simulink model "Offline_DataImport_AND_ECGAnalysis_AND_SCGAnalysis"  (R2020b)
settings: Solver=FixedStepDiscrete  StartTime=0.0  StopTime=param_sim_time  FixedStep=1/fs  MaxStep=1/fs  RelTol=1e-3
undefined symbols (not defined in the file): analyses, fdesignblkfcn, fs, gcbh, param_tot_samples
libraries: dspstat3 x1
(part 5 of 5)

== matlab function Offline_DataImport_AND_ECGAnalysis_AND_SCGAnalysis/SCG Analysis/Enabled SCG Analysis Subsystem/Signal Generation/3D Projections/SCG xyz Average Cycle/Average SCGxyz Cycle Calculator ==
  data: r_pos input; scgxyz input; scgxyz_avgcycle output size=[3*fs 3]
function scgxyz_avgcycle  = slk_avg_scgxyz_cycle_calculator(r_pos,scgxyz)
% Simulink function to return the average x,y, and z cycles of the SCG.

% INPUTS:
% r_pos = index positions of the R peaks of the ecg.
% scgxyz = matrix of size [length_scg 3] with the (normally pre-processed) SCG
%          x,y, and z components. The first column corresponds to SCGx, the second
%          to SCGy and the third to SCGz.

% OUTPUT:
% avg_scg_xyz = matrix of size [min_rr 3] with the average SCG cycles of
%               the x,y, and z components. The first column corresponds to SCGx, the second
%               to SCGy and the third to SCGz 


% Calculating number of cycles to be considered in averaging (considered_cycles).
rr_min = min(diff(r_pos)); % Shortest cycle length - all the cycles will but cut down to this length.

if length(scgxyz) > r_pos(end) + rr_min
    considered_cycles = length(r_pos);
else
    considered_cycles = length(r_pos) - 1;
end

scg_x_cycles = zeros(rr_min,considered_cycles);
scg_y_cycles = zeros(rr_min,considered_cycles);
scg_z_cycles = zeros(rr_min,considered_cycles);

fig_scg_average_cycles = figure;

% Isolating and plotting each cycle
for i = 1:considered_cycles
    figure(fig_scg_average_cycles);
    scg_x_cycles(:,i) = scgxyz(r_pos(i):r_pos(i) + rr_min - 1,1);
    scg_y_cycles(:,i) = scgxyz(r_pos(i):r_pos(i) + rr_min - 1,2);
    scg_z_cycles(:,i) = scgxyz(r_pos(i):r_pos(i) + rr_min - 1,3);
    
    % Plotting
    subplot(3,1,1); plot(scg_x_cycles(:,i),'b'); hold on;
    subplot(3,1,2); plot(scg_y_cycles(:,i),'b'); hold on;
    subplot(3,1,3); plot(scg_z_cycles(:,i),'b'); hold on;
end

% Calculating average cycle
avg_scg_x = mean(scg_x_cycles,2);
avg_scg_y = mean(scg_y_cycles,2);
avg_scg_z = mean(scg_z_cycles,2);

% Plotting the average cycle
subplot(3,1,1); plot(avg_scg_x,'k','LineWidth',2); title('Average SCG x'); box off;
subplot(3,1,2); plot(avg_scg_y,'k','LineWidth',2); title('Average SCG y'); ylabel('Amplitude (mg)'); box off;
subplot(3,1,3); plot(avg_scg_z,'k','LineWidth',2); title('Average SCG z'); xlabel('Time (msec)'); box off;

scgxyz_avgcycle = [avg_scg_x avg_scg_y avg_scg_z];
end

== matlab function Offline_DataImport_AND_ECGAnalysis_AND_SCGAnalysis/SCG Analysis/Enabled SCG Analysis Subsystem/Signal Generation/3D Projections/SCG xyz Average Cycle/Min RR Calculator ==
  data: r_pos input; min_rr output size=[1]
function min_rr  = slk_min_rr_calculator(r_pos)
% Simulink function to calculate the shortest RR interval from a sequence
% of R peak inputs.

% INPUTS:
% r_pos = index positions of the R peaks of the ecg.

% OUTPUT:
% min_rr = minimum RR interval.

if r_pos % Only enter the function if a valid r_pos sequence is passed to it.
    min_rr = min(diff(r_pos)); % Shortest cycle length - all the cycles will but cut down to this length.
else
    min_rr = 0;
end
end

== matlab function Offline_DataImport_AND_ECGAnalysis_AND_SCGAnalysis/SCG Analysis/Enabled SCG Analysis Subsystem/Anisotropy Characterization/Average Max Diameter//Volume Calculator/Wrapped Average Max Diameter//Volume Calculator ==
  data: fs input size=[1]; r_pos input size=[4*ceil(param_sim_time) 1]; scg_xyz input size=[param_tot_samples 3]; avg_max_diameter_over_volume output size=[1]
function avg_max_diameter_over_volume = wrapped_anisotropy_calculator_avg_max_diameter_over_volume(fs,r_pos,scg_xyz) 
avg_max_diameter_over_volume=-1; % Pre-Initialization.
coder.extrinsic('anisotropy_calculator_avg_max_diameter_over_volume');
avg_max_diameter_over_volume = anisotropy_calculator_avg_max_diameter_over_volume(fs,r_pos,scg_xyz); 
end

== matlab function Offline_DataImport_AND_ECGAnalysis_AND_SCGAnalysis/SCG Analysis/Enabled SCG Analysis Subsystem/Anisotropy Characterization/Average Cycle Max Diameter//Volume Calculator/Wrapped Average Cycle Max Diameter//Volume Calculator ==
  data: avg_s1_xyz input size=[0.2*fs 3]; avg_cycle_max_diameter_over_volume output size=[1]
function avg_cycle_max_diameter_over_volume = wrapped_anisotropy_calculator_avg_cycle_max_diameter_over_vol(avg_s1_xyz) 
avg_cycle_max_diameter_over_volume = -1; % Pre-Initialization.
coder.extrinsic('anisotropy_calculator_avg_cycle_max_diameter_over_volume');
avg_cycle_max_diameter_over_volume = anisotropy_calculator_avg_cycle_max_diameter_over_volume(avg_s1_xyz); 
end

== matlab function Offline_DataImport_AND_ECGAnalysis_AND_SCGAnalysis/SCG Analysis/Enabled SCG Analysis Subsystem/Anisotropy Characterization/Average Cycle Max Diameter//Volume Calculator/SCG xyz Average Cycle/Average SCGxyz Cycle Calculator ==
  data: r_pos input; scgxyz input; scgxyz_avgcycle output size=[3*fs 3]
function scgxyz_avgcycle  = slk_avg_scgxyz_cycle_calculator(r_pos,scgxyz)
% Simulink function to return the average x,y, and z cycles of the SCG.

% INPUTS:
% r_pos = index positions of the R peaks of the ecg.
% scgxyz = matrix of size [length_scg 3] with the (normally pre-processed) SCG
%          x,y, and z components. The first column corresponds to SCGx, the second
%          to SCGy and the third to SCGz.

% OUTPUT:
% avg_scg_xyz = matrix of size [min_rr 3] with the average SCG cycles of
%               the x,y, and z components. The first column corresponds to SCGx, the second
%               to SCGy and the third to SCGz 


% Calculating number of cycles to be considered in averaging (considered_cycles).
rr_min = min(diff(r_pos)); % Shortest cycle length - all the cycles will but cut down to this length.

if length(scgxyz) > r_pos(end) + rr_min
    considered_cycles = length(r_pos);
else
    considered_cycles = length(r_pos) - 1;
end

scg_x_cycles = zeros(rr_min,considered_cycles);
scg_y_cycles = zeros(rr_min,considered_cycles);
scg_z_cycles = zeros(rr_min,considered_cycles);

% fig_scg_average_cycles = figure;

% Isolating and plotting each cycle
for i = 1:considered_cycles
%     figure(fig_scg_average_cycles);
    scg_x_cycles(:,i) = scgxyz(r_pos(i):r_pos(i) + rr_min - 1,1);
    scg_y_cycles(:,i) = scgxyz(r_pos(i):r_pos(i) + rr_min - 1,2);
    scg_z_cycles(:,i) = scgxyz(r_pos(i):r_pos(i) + rr_min - 1,3);
    
    % Plotting
%     subplot(3,1,1); plot(scg_x_cycles(:,i),'b'); hold on;
%     subplot(3,1,2); plot(scg_y_cycles(:,i),'b'); hold on;
%     subplot(3,1,3); plot(scg_z_cycles(:,i),'b'); hold on;
end

% Calculating average cycle
avg_scg_x = mean(scg_x_cycles,2);
avg_scg_y = mean(scg_y_cycles,2);
avg_scg_z = mean(scg_z_cycles,2);

% Plotting the average cycle
% subplot(3,1,1); plot(avg_scg_x,'k','LineWidth',2); title('Average SCG x'); box off;
% subplot(3,1,2); plot(avg_scg_y,'k','LineWidth',2); title('Average SCG y'); ylabel('Amplitude (mg)'); box off;
% subplot(3,1,3); plot(avg_scg_z,'k','LineWidth',2); title('Average SCG z'); xlabel('Time (msec)'); box off;

scgxyz_avgcycle = [avg_scg_x avg_scg_y avg_scg_z];
end

== matlab function Offline_DataImport_AND_ECGAnalysis_AND_SCGAnalysis/SCG Analysis/Enabled SCG Analysis Subsystem/Anisotropy Characterization/Average Cycle Max Diameter//Volume Calculator/SCG xyz Average Cycle/Min RR Calculator ==
  data: r_pos input; min_rr output size=[1]
function min_rr  = slk_min_rr_calculator(r_pos)
% Simulink function to calculate the shortest RR interval from a sequence
% of R peak inputs.

% INPUTS:
% r_pos = index positions of the R peaks of the ecg.

% OUTPUT:
% min_rr = minimum RR interval.

if r_pos % Only enter the function if a valid r_pos sequence is passed to it.
    min_rr = min(diff(r_pos)); % Shortest cycle length - all the cycles will but cut down to this length.
else
    min_rr = 0;
end
end

== matlab function Offline_DataImport_AND_ECGAnalysis_AND_SCGAnalysis/SCG Analysis/Enabled SCG Analysis Subsystem/Anisotropy Characterization/Average Max//Min Diameter Calculator/Wrapped Average Max//Min Diameters Calculator ==
  data: fs input size=[1]; r_pos input size=[4*ceil(param_sim_time) 1]; scg_xyz input size=[param_tot_samples 3]; avg_max_over_min_diameters output size=[1]
function avg_max_over_min_diameters = wrapped_anisotropy_calculator_avg_max_over_min_diameters(fs,r_pos,scg_xyz) 
avg_max_over_min_diameters = -1; % Pre-Initialization.
coder.extrinsic('anisotropy_calculator_avg_max_over_min_diameters');
avg_max_over_min_diameters = anisotropy_calculator_avg_max_over_min_diameters(fs,r_pos,scg_xyz); 
end

== matlab function Offline_DataImport_AND_ECGAnalysis_AND_SCGAnalysis/SCG Analysis/Enabled SCG Analysis Subsystem/Anisotropy Characterization/Average Cycle Max//Min Diameter Calculator/SCG xyz Average Cycle/Average SCGxyz Cycle Calculator ==
  data: r_pos input; scgxyz input; scgxyz_avgcycle output size=[3*fs 3]
function scgxyz_avgcycle  = slk_avg_scgxyz_cycle_calculator(r_pos,scgxyz)
% Simulink function to return the average x,y, and z cycles of the SCG.

% INPUTS:
% r_pos = index positions of the R peaks of the ecg.
% scgxyz = matrix of size [length_scg 3] with the (normally pre-processed) SCG
%          x,y, and z components. The first column corresponds to SCGx, the second
%          to SCGy and the third to SCGz.

% OUTPUT:
% avg_scg_xyz = matrix of size [min_rr 3] with the average SCG cycles of
%               the x,y, and z components. The first column corresponds to SCGx, the second
%               to SCGy and the third to SCGz 


% Calculating number of cycles to be considered in averaging (considered_cycles).
rr_min = min(diff(r_pos)); % Shortest cycle length - all the cycles will but cut down to this length.

if length(scgxyz) > r_pos(end) + rr_min
    considered_cycles = length(r_pos);
else
    considered_cycles = length(r_pos) - 1;
end

scg_x_cycles = zeros(rr_min,considered_cycles);
scg_y_cycles = zeros(rr_min,considered_cycles);
scg_z_cycles = zeros(rr_min,considered_cycles);

% fig_scg_average_cycles = figure;

% Isolating and plotting each cycle
for i = 1:considered_cycles
%     figure(fig_scg_average_cycles);
    scg_x_cycles(:,i) = scgxyz(r_pos(i):r_pos(i) + rr_min - 1,1);
    scg_y_cycles(:,i) = scgxyz(r_pos(i):r_pos(i) + rr_min - 1,2);
    scg_z_cycles(:,i) = scgxyz(r_pos(i):r_pos(i) + rr_min - 1,3);
    
    % Plotting
%     subplot(3,1,1); plot(scg_x_cycles(:,i),'b'); hold on;
%     subplot(3,1,2); plot(scg_y_cycles(:,i),'b'); hold on;
%     subplot(3,1,3); plot(scg_z_cycles(:,i),'b'); hold on;
end

% Calculating average cycle
avg_scg_x = mean(scg_x_cycles,2);
avg_scg_y = mean(scg_y_cycles,2);
avg_scg_z = mean(scg_z_cycles,2);

% Plotting the average cycle
% subplot(3,1,1); plot(avg_scg_x,'k','LineWidth',2); title('Average SCG x'); box off;
% subplot(3,1,2); plot(avg_scg_y,'k','LineWidth',2); title('Average SCG y'); ylabel('Amplitude (mg)'); box off;
% subplot(3,1,3); plot(avg_scg_z,'k','LineWidth',2); title('Average SCG z'); xlabel('Time (msec)'); box off;

scgxyz_avgcycle = [avg_scg_x avg_scg_y avg_scg_z];
end

== matlab function Offline_DataImport_AND_ECGAnalysis_AND_SCGAnalysis/SCG Analysis/Enabled SCG Analysis Subsystem/Anisotropy Characterization/Average Cycle Max//Min Diameter Calculator/SCG xyz Average Cycle/Min RR Calculator ==
  data: r_pos input; min_rr output size=[1]
function min_rr  = slk_min_rr_calculator(r_pos)
% Simulink function to calculate the shortest RR interval from a sequence
% of R peak inputs.

% INPUTS:
% r_pos = index positions of the R peaks of the ecg.

% OUTPUT:
% min_rr = minimum RR interval.

if r_pos % Only enter the function if a valid r_pos sequence is passed to it.
    min_rr = min(diff(r_pos)); % Shortest cycle length - all the cycles will but cut down to this length.
else
    min_rr = 0;
end
end

== matlab function Offline_DataImport_AND_ECGAnalysis_AND_SCGAnalysis/ECG Analysis/Enabled ECG Analysis Subsystem/Coherent Segmentation/Slk Coherent Segmentation Function ==
  data: ecg_p input size=[4*ceil(param_sim_time) 1]; coherent_ecg_pqrst output size=[4*ceil(param_sim_time) 5]; ecg_q input size=[4*ceil(param_sim_time) 1]; ecg_r input size=[4*ceil(param_sim_time) 1]; ecg_s input size=[4*ceil(param_sim_time) 1]; ecg_t input size=[4*ceil(param_sim_time) 1]; num_cycles output size=1
function [coherent_ecg_pqrst, num_cycles] = slk_coherent_segmentation(ecg_p, ecg_q, ecg_r, ecg_s, ecg_t)
% Function to associate the detected PQRST peaks to each other in a
% coherent way. The function will produce an output 'coherent_ecg_pqrst' of
% size [num_cycles x 5]. The 5 corresponds to the 5 fiducial points (PQRST
% peaks). num_cycles is the number of detected R peaks (heart cycles). The
% first column of coherent_ecg_prqst corresponds to the detected P waves,
% where the row corresponds to that cycle number. If a P wave couldnt be
% detected for that cycle, it is replaced with 'Nan'.


if ecg_r % Only go into the function if a valid ecg R peak sequence is passed to it.
    
    % Preinitialization.
    coherent_ecg_p = zeros(length(ecg_r),1);
    coherent_ecg_q = zeros(length(ecg_r),1);
    coherent_ecg_r = zeros(length(ecg_r),1);
    coherent_ecg_s = zeros(length(ecg_r),1);
    coherent_ecg_t = zeros(length(ecg_r),1);
        
    %% First Cycle.
    
    % P Wave.
    temp = ecg_p(find(ecg_p < ecg_r(1)));
    if isempty(temp)
        coherent_ecg_p(1) = nan;
        temp = [];
    else
        coherent_ecg_p(1) = temp;
    end
    
    % Q Wave.
    temp = ecg_p(find(ecg_q < ecg_r(1)));
    if isempty(temp)
        coherent_ecg_q(1) = nan;
        temp = [];
    else
        coherent_ecg_q(1) = temp;
    end
    
    % R Wave.
    coherent_ecg_r(1) = ecg_r(1);
    
    % S Wave.
    temp = ecg_s(find(ecg_s > ecg_r(1) & ecg_s < ecg_r(2)));
    if isempty(temp)
        coherent_ecg_s(1) = nan;
        temp = [];
    else
        coherent_ecg_s(1) = temp;
    end
    
    % T Wave.
    temp = ecg_t(find(ecg_t > ecg_r(1) & ecg_t < ecg_r(2)));
    if isempty(temp)
        coherent_ecg_t(1) = nan;
        temp = [];
    else
        coherent_ecg_t(1) = temp;
    end
    
    %% Cycle 2:End-1.
    for i = 2:length(ecg_r)-1
        
        % P Wave.
        temp = ecg_p(find(ecg_p > ecg_r(i-1) & ecg_p < ecg_r(i)));
        if isempty(temp) || length(temp) > 1
            coherent_ecg_p(i) = nan;
            temp = [];
        else
            coherent_ecg_p(i) = temp;
        end
        
        % Q Wave.
        temp = ecg_q(find(ecg_q > ecg_r(i-1) & ecg_q < ecg_r(i)));
        if isempty(temp) || length(temp) > 1
            coherent_ecg_q(i) = nan;
            temp = [];
        else
            coherent_ecg_q(i) = temp;
        end
        
        % R Wave.
        coherent_ecg_r(i) = ecg_r(i);
        
        % S Wave.
        temp = ecg_s(find(ecg_s > ecg_r(i) & ecg_s < ecg_r(i+1)));
        if isempty(temp) || length(temp) > 1
            coherent_ecg_s(i) = nan;
            temp = [];
        else
            coherent_ecg_s(i) = temp;
        end
        
        % T Wave.
        temp = ecg_t(find(ecg_t > ecg_r(i) & ecg_t < ecg_r(i+1)));
        if isempty(temp) || length(temp) > 1
            coherent_ecg_t(i) = nan;
            temp = [];
        else
            coherent_ecg_t(i) = temp;
        end
    end
    
    %% Last Cycle.
    
    % P Wave.
    temp = ecg_p(find(ecg_p > ecg_r(end-1) & ecg_p < ecg_r(end)));
    if isempty(temp) || length(temp) > 1
        coherent_ecg_p(length(ecg_r)) = nan;
        temp = [];
    else
        coherent_ecg_p(length(ecg_r)) = temp;
    end
    
    % Q Wave.
    temp = ecg_q(find(ecg_q > ecg_r(end-1) & ecg_q < ecg_r(end)));
    if isempty(temp) || length(temp) > 1
        coherent_ecg_q(length(ecg_r)) = nan;
        temp = [];
    else
        coherent_ecg_q(length(ecg_r)) = temp;
    end
    
    % R Wave.
    coherent_ecg_r(length(ecg_r)) = ecg_r(length(ecg_r));
    
    % S Wave.
    temp = ecg_s(find(ecg_s > ecg_r(1) & ecg_s < ecg_r(2)));
    if isempty(temp) || length(temp) > 1
        coherent_ecg_s(length(ecg_r)) = nan;
        temp = [];
    else
        coherent_ecg_s(length(ecg_r)) = temp;
    end
    
    % T Wave.
    temp = ecg_t(find(ecg_t > ecg_r(1) & ecg_t < ecg_r(2)));
    if isempty(temp) || length(temp) > 1
        coherent_ecg_t(length(ecg_r)) = nan;
        temp = [];
    else
        coherent_ecg_t(length(ecg_r)) = temp;
    end
    
    coherent_ecg_pqrst = [coherent_ecg_p coherent_ecg_q coherent_ecg_r coherent_ecg_s coherent_ecg_t];
    num_cycles = length(coherent_ecg_r);  
    
else
    
    coherent_ecg_pqrst = [];
    num_cycles = 0;
end
end

== matlab function Offline_DataImport_AND_ECGAnalysis_AND_SCGAnalysis/SCG Analysis/Enabled SCG Analysis Subsystem/Anisotropy Characterization/Average Max//Median Diameter Calculator/Wrapped Average Max//Median Diameter Calculator ==
  data: fs input size=[1]; r_pos input size=[4*ceil(param_sim_time) 1]; scg_xyz input size=[param_tot_samples 3]; avg_max_over_median_diameter output size=[1]
function avg_max_over_median_diameter = wrapped_anisotropy_calculator_avg_max_over_median_diameter(fs,r_pos,scg_xyz) 
avg_max_over_median_diameter = -1; % Pre-Initialization.
coder.extrinsic('anisotropy_calculator_avg_max_over_median_diameter');
avg_max_over_median_diameter = anisotropy_calculator_avg_max_over_median_diameter(fs,r_pos,scg_xyz); 
end

== matlab function Offline_DataImport_AND_ECGAnalysis_AND_SCGAnalysis/SCG Analysis/Enabled SCG Analysis Subsystem/Anisotropy Characterization/Average Cycle Max//Min Diameter Calculator/Wrapped Average Cycle Max//Min Diameters Calculator ==
  data: avg_s1_xyz input size=[0.2*fs 3]; avg_cycle_max_over_min_diameters output size=[1]
function avg_cycle_max_over_min_diameters = wrapped_anisotropy_calculator_avg_cycle_max_over_min_diameters(avg_s1_xyz) 
avg_cycle_max_over_min_diameters = -1; % Pre-Initialization.
coder.extrinsic('anisotropy_calculator_avg_cycle_max_over_min_diameters');
avg_cycle_max_over_min_diameters = anisotropy_calculator_avg_cycle_max_over_min_diameters(avg_s1_xyz); 
end

== matlab function Offline_DataImport_AND_ECGAnalysis_AND_SCGAnalysis/SCG Analysis/Enabled SCG Analysis Subsystem/Anisotropy Characterization/Average Cycle Max//Median Diameter Calculator/SCG xyz Average Cycle/Average SCGxyz Cycle Calculator ==
  data: r_pos input; scgxyz input; scgxyz_avgcycle output size=[3*fs 3]
function scgxyz_avgcycle  = slk_avg_scgxyz_cycle_calculator(r_pos,scgxyz)
% Simulink function to return the average x,y, and z cycles of the SCG.

% INPUTS:
% r_pos = index positions of the R peaks of the ecg.
% scgxyz = matrix of size [length_scg 3] with the (normally pre-processed) SCG
%          x,y, and z components. The first column corresponds to SCGx, the second
%          to SCGy and the third to SCGz.

% OUTPUT:
% avg_scg_xyz = matrix of size [min_rr 3] with the average SCG cycles of
%               the x,y, and z components. The first column corresponds to SCGx, the second
%               to SCGy and the third to SCGz 


% Calculating number of cycles to be considered in averaging (considered_cycles).
rr_min = min(diff(r_pos)); % Shortest cycle length - all the cycles will but cut down to this length.

if length(scgxyz) > r_pos(end) + rr_min
    considered_cycles = length(r_pos);
else
    considered_cycles = length(r_pos) - 1;
end

scg_x_cycles = zeros(rr_min,considered_cycles);
scg_y_cycles = zeros(rr_min,considered_cycles);
scg_z_cycles = zeros(rr_min,considered_cycles);

% fig_scg_average_cycles = figure;

% Isolating and plotting each cycle
for i = 1:considered_cycles
%     figure(fig_scg_average_cycles);
    scg_x_cycles(:,i) = scgxyz(r_pos(i):r_pos(i) + rr_min - 1,1);
    scg_y_cycles(:,i) = scgxyz(r_pos(i):r_pos(i) + rr_min - 1,2);
    scg_z_cycles(:,i) = scgxyz(r_pos(i):r_pos(i) + rr_min - 1,3);
    
    % Plotting
%     subplot(3,1,1); plot(scg_x_cycles(:,i),'b'); hold on;
%     subplot(3,1,2); plot(scg_y_cycles(:,i),'b'); hold on;
%     subplot(3,1,3); plot(scg_z_cycles(:,i),'b'); hold on;
end

% Calculating average cycle
avg_scg_x = mean(scg_x_cycles,2);
avg_scg_y = mean(scg_y_cycles,2);
avg_scg_z = mean(scg_z_cycles,2);

% Plotting the average cycle
% subplot(3,1,1); plot(avg_scg_x,'k','LineWidth',2); title('Average SCG x'); box off;
% subplot(3,1,2); plot(avg_scg_y,'k','LineWidth',2); title('Average SCG y'); ylabel('Amplitude (mg)'); box off;
% subplot(3,1,3); plot(avg_scg_z,'k','LineWidth',2); title('Average SCG z'); xlabel('Time (msec)'); box off;

scgxyz_avgcycle = [avg_scg_x avg_scg_y avg_scg_z];
end

== matlab function Offline_DataImport_AND_ECGAnalysis_AND_SCGAnalysis/SCG Analysis/Enabled SCG Analysis Subsystem/Anisotropy Characterization/Average Cycle Max//Median Diameter Calculator/SCG xyz Average Cycle/Min RR Calculator ==
  data: r_pos input; min_rr output size=[1]
function min_rr  = slk_min_rr_calculator(r_pos)
% Simulink function to calculate the shortest RR interval from a sequence
% of R peak inputs.

% INPUTS:
% r_pos = index positions of the R peaks of the ecg.

% OUTPUT:
% min_rr = minimum RR interval.

if r_pos % Only enter the function if a valid r_pos sequence is passed to it.
    min_rr = min(diff(r_pos)); % Shortest cycle length - all the cycles will but cut down to this length.
else
    min_rr = 0;
end
end

== matlab function Offline_DataImport_AND_ECGAnalysis_AND_SCGAnalysis/SCG Analysis/Enabled SCG Analysis Subsystem/Anisotropy Characterization/Average Cycle Max//Median Diameter Calculator/Wrapped Average Cycle Max//Median Diameter Calculator ==
  data: avg_s1_xyz input size=[0.2*fs 3]; avg_cycle_max_over_median_diameter output size=[1]
function avg_cycle_max_over_median_diameter = wrapped_anisotropy_calculator_avg_cycle_max_over_med_diameter(avg_s1_xyz) 
avg_cycle_max_over_median_diameter = -1; % Pre-Initialization.
coder.extrinsic('anisotropy_calculator_avg_cycle_max_over_median_diameter');
avg_cycle_max_over_median_diameter = anisotropy_calculator_avg_cycle_max_over_median_diameter(avg_s1_xyz); 
end

== matlab function Offline_DataImport_AND_ECGAnalysis_AND_SCGAnalysis/ECG Analysis/Enabled ECG Analysis Subsystem/Plotting ==
  data: coherent_ecg_pqrst input size=[4*ceil(param_sim_time) 5]; preprocessed_ecg input size=[param_tot_samples 1]; fs input size=[1]
function slk_wrapped_plotting_ecg_pqrst(coherent_ecg_pqrst, preprocessed_ecg, fs)
    
coder.extrinsic('plotting_ecg_pqrst');

if coherent_ecg_pqrst(:,3) % Only go into the function if a valid ecg R peak sequence is passed to it.
    plotting_ecg_pqrst(coherent_ecg_pqrst, preprocessed_ecg, fs)
end

end

== matlab function Offline_DataImport_AND_ECGAnalysis_AND_SCGAnalysis/ECG Preprocessing/Enabled ECG Preprocessing Subsystem/Plotting ==
  data: preprocessed_ecg input size=[param_tot_samples 1]; raw_ecg input size=[param_tot_samples 1]; fs input size=[1]
function slk_wrapped_plotting_preprocessed_ecg(preprocessed_ecg, raw_ecg, fs)
    
coder.extrinsic('plotting_preprocessed_ecg');

if preprocessed_ecg % Only go into the function if a valid ecg R peak sequence is passed to it.
    plotting_preprocessed_ecg(preprocessed_ecg, raw_ecg, fs)
end

end

== matlab function Offline_DataImport_AND_ECGAnalysis_AND_SCGAnalysis/ECG Analysis/Enabled ECG Analysis Subsystem/Ectopic Correction/Ectopic Correction ==
  data: fs input; max_hr input; max_rr_dev input; r_pos input size=[4*ceil(param_sim_time) 1]; corrected_r_pos output size=[4*ceil(param_sim_time) 1]
function corrected_r_pos = slk_ectopic_correction(fs, max_hr, max_rr_dev, r_pos)

if r_pos % Only run if a series of R peaks are passed.
    
    corrected_r_pos = r_pos;
    
    rr = diff(r_pos); % RR interval calculation.
    
    %% Part 1 - Identification of Cycles over the Maximum Heart Rate.
    max_rr_sec = 1/(max_hr/60); % In sec.
    max_rr_samples = max_rr_sec*fs; % In samples.
    
    tachogram = 60./(rr/fs); % Tachogram calculation (in bpm).
    
    % Plotting the tachogram.
    fig_tachogram = figure;
    plot(r_pos(1:end-1)/fs,tachogram); title('Tachogram'); xlabel('R Time (sec)'); ylabel('Heart Rate (bpm)'); box off; hold on;
    line([0 r_pos(end-1)/fs],[max_hr max_hr],'Color','red','LineStyle','--'); hold on
    
    % Identifying the ectopies faster than the Maximum Heart Rate threshold and labelling them as 'nan'.
    ectopies_1 = find(rr < max_rr_samples);
    rr(ectopies_1) = nan;
    r_pos(ectopies_1 + 1) = nan;
    
    %% Part 2 - Identification of Cycles over the RR Deviation Threshold.    
    % Evaluating the adaptive RR deviation threshold (a 7-cycle moving median). The detected ectopies of part 1 do not compute for this moving median.
    plot_thr = 60./(movmedian(rr,7,'omitnan')/fs) + max_rr_dev; % The threshold to be plotted on the tachogram (in bpm).
    thr = fs./(plot_thr/60); % The equivalent threshold in samples - to be compared against the calculated RR intervals.
    
    % Plotting the adaptive threshold on the tachogram.
    plot(r_pos(1:end-1)/fs,plot_thr,'r--'); hold on;
    
    % Identifying Ectopies
    ectopies_2 = find(thr - rr > 0 );
    
    %% Part 3 - Labelling and removing the detected ectopies.

    ectopies = [ectopies_1; ectopies_2];
    ectopies = sort(ectopies);
    
    plot(r_pos(ectopies)/fs,tachogram(ectopies),'ro'); hold on; 
    corrected_r_pos(ectopies) = [];
   
else
    corrected_r_pos = r_pos;
end

end

== matlab function Offline_DataImport_AND_ECGAnalysis_AND_SCGAnalysis/SCG Preprocessing/Enabled SCG Preprocessing Subsystem/Plotting ==
  data: preprocessed_scg_xyz input size=[param_tot_samples 3]; raw_scg_xyz input size=[param_tot_samples 3]; fs input size=[1]
function slk_wrapped_plotting_preprocessed_scg_xyz(preprocessed_scg_xyz, raw_scg_xyz, fs)
    
coder.extrinsic('plotting_preprocessed_scg_xyz');

if preprocessed_scg_xyz(:,1) % Only go into the function if a valid ecg R peak sequence is passed to it.
    plotting_preprocessed_scg_xyz(preprocessed_scg_xyz, raw_scg_xyz, fs);
end

end

== matlab function Offline_DataImport_AND_ECGAnalysis_AND_SCGAnalysis/ECG Analysis/Enabled ECG Analysis Subsystem/P,Q,R,S,T Detection/Wrapped BioSigKit ECG PQRST Detection ==
  data: ecg_p output size=[4*ceil(param_sim_time) 1]; ecg_q output size=[4*ceil(param_sim_time) 1]; ecg_r output size=[4*ceil(param_sim_time) 1]; ecg_s output size=[4*ceil(param_sim_time) 1]; ecg_t output size=[4*ceil(param_sim_time) 1]; fs input; preprocessed_ecg input; ecg_algo input
function [ecg_p, ecg_q, ecg_r, ecg_s, ecg_t] = slk_wrapped_BioSigKit_ECG_Detection(fs, preprocessed_ecg, ecg_algo)

% This function is split in two parts out of necessity - (Simulink is kind of dumb).
% The first part counts how many detected P,Q,R,S, and T waves there are according to the BioSigKit method.
% With these numbers we can pre-initialize the size of the vectors holding the sample positions of these P,Q,R,S, and T waves which are then
% identified using a second identical use of the BioSigKit detection method.

coder.extrinsic('BioSigKit_ECG_Count_Detection');
coder.extrinsic('BioSigKit_ECG_Peak_Detection');

if preprocessed_ecg % The function is only run if a non-zero signal is passed to it.
    %% Part 1 - P,Q,R,S,T Count
    num_p = -1; % Pre-Initialization.
    num_q = -1;
    num_r = -1;
    num_s = -1;
    num_t = -1;
    
    [num_p, num_q, num_r, num_s, num_t] = BioSigKit_ECG_Count_Detection(fs,preprocessed_ecg, ecg_algo);
    
    %% Part 2 - P,Q,R,S,T Peak Identification
    ecg_p = zeros(num_p,1); % Pre-Initialization.
    ecg_q = zeros(num_q,1);
    ecg_r = zeros(num_r,1);
    ecg_s = zeros(num_s,1);
    ecg_t = zeros(num_t,1);
    
    % Performing the detection according to the desired detection algorithm.
    if ecg_algo == 1  || ecg_algo == 2 || ecg_algo == 3
        
        [~, ~, ecg_r(1:num_r), ~, ~] = BioSigKit_ECG_Peak_Detection(fs,preprocessed_ecg, ecg_algo);
        ecg_p = nan; ecg_q = nan; ecg_s = nan; ecg_t = nan;
        
    elseif ecg_algo == 4
        
        [~, ecg_q(1:num_q), ecg_r(1:num_r), ecg_s(1:num_s), ecg_t(1:num_t)] = BioSigKit_ECG_Peak_Detection(fs,preprocessed_ecg, ecg_algo);
        ecg_p = nan;
        
    elseif ecg_algo == 5
        
        [ecg_p(1:num_p), ecg_q(1:num_q), ecg_r(1:num_r), ecg_s(1:num_s), ecg_t(1:num_t)] = BioSigKit_ECG_Peak_Detection(fs,preprocessed_ecg, ecg_algo);
        
    end
        
else % If there's no input - pass an empty output.
    
    ecg_p = [];
    ecg_q = [];
    ecg_r = [];
    ecg_s = [];
    ecg_t = [];
    
end

== matlab function Offline_DataImport_AND_ECGAnalysis_AND_SCGAnalysis/SCG Analysis/Enabled SCG Analysis Subsystem/Signal Generation/2D Mod Average Cycle/Average 2DMod Cycle Calculator ==
  data: r_pos input; signal input; avg_cycle output size=[param_tot_samples 1]
function avg_cycle  = slk_avg_cycle_calculator(r_pos, signal)
% Simulink function to return the average cycle of an arbitraty signal input.

% INPUTS:
% r_pos = index positions of the R peaks of the ecg.
% signal = arbitrary input signal.

% OUTPUT:
% avg_cycle = averaged cycle of arbitrary input signal.


% Calculating number of cycles to be considered in averaging
rr_min = min(diff(r_pos)); % Shortest cycle length - all the cycles will but cut down to this length.

if length(signal) > r_pos(end) + rr_min
    considered_cycles = length(r_pos);
else
    considered_cycles = length(r_pos) - 1;
end

signal_cycles = zeros(rr_min,considered_cycles);

fig_average_cycle = figure;

% Isolating and plotting each cycle
for i = 1:considered_cycles
    signal_cycles(:,i) = signal(r_pos(i):r_pos(i) + rr_min - 1,1);
    figure(fig_average_cycle); plot(signal_cycles(:,i),'b'); hold on
end

% Calculating average cycle
avg_cycle = mean(signal_cycles,2);

% Plotting the average cycle
figure(fig_average_cycle); plot(avg_cycle,'k','LineWidth',2); title('Average Cycle'); xlabel('Time (msec)'); ylabel('Acceleration (mg)'); box off;
title('2D Modulus')
end

== matlab function Offline_DataImport_AND_ECGAnalysis_AND_SCGAnalysis/SCG Analysis/Enabled SCG Analysis Subsystem/Signal Generation/3D Mod Average Cycle/Average 3DMod Cycle Calculator ==
  data: r_pos input; signal input; avg_cycle output size=[param_tot_samples 1]
function avg_cycle  = slk_avg_cycle_calculator(r_pos, signal)
% Simulink function to return the average cycle of an arbitraty signal input.

% INPUTS:
% r_pos = index positions of the R peaks of the ecg.
% signal = arbitrary input signal.

% OUTPUT:
% avg_cycle = averaged cycle of arbitrary input signal.


% Calculating number of cycles to be considered in averaging
rr_min = min(diff(r_pos)); % Shortest cycle length - all the cycles will but cut down to this length.

if length(signal) > r_pos(end) + rr_min
    considered_cycles = length(r_pos);
else
    considered_cycles = length(r_pos) - 1;
end

signal_cycles = zeros(rr_min,considered_cycles);

fig_average_cycle = figure;

% Isolating and plotting each cycle
for i = 1:considered_cycles
    figure(fig_average_cycle);
    signal_cycles(:,i) = signal(r_pos(i):r_pos(i) + rr_min - 1,1);
    plot(signal_cycles(:,i),'b'); hold on
end

% Calculating average cycle
avg_cycle = mean(signal_cycles,2);

% Plotting the average cycle
plot(avg_cycle,'k','LineWidth',2); title('Average Cycle'); xlabel('Time (msec)'); ylabel('Acceleration (mg)'); box off;
title('3D Modulus')
end

== matlab function Offline_DataImport_AND_ECGAnalysis_AND_SCGAnalysis/SCG Analysis/Enabled SCG Analysis Subsystem/Signal Generation/3D Projections/MATLAB Function ==
  data: scg_xyz input; el_scg input size=[1]; projection output size=[param_tot_samples 1]; az_scg input size=[1]
function projection = slk_axis_projection(scg_xyz, el_scg, az_scg)

el_mat = el_scg;
az_mat = -1*az_scg;

[xhat_mat, yhat_mat, zhat_mat] = sph2cart(az_mat*pi/180,el_mat*pi/180,1);
% Converting to the SCG convention reference frame (this depends on the accelerometer and its placement orientation! - they should be such that they match the conventional SCG reference frame).
xhat_scg = xhat_mat;
yhat_scg = zhat_mat;
zhat_scg = -1*yhat_mat;

projection_axis = [xhat_scg yhat_scg zhat_scg];
    
projection = zeros(size(scg_xyz,1),1);
    
for i=1:size(scg_xyz,1)
    
    projection(i) = dot(scg_xyz(i,:),projection_axis);
    
end

figure;
ax = [0 0 0 0];

ax(1) = subplot(4,1,1); plot(scg_xyz(:,1),'b'); title('x'); box off; ylabel('Acceleration (mg)');
ax(2) = subplot(4,1,2); plot(scg_xyz(:,2),'b'); title('y'); box off; ylabel('Acceleration (mg)');
ax(3) = subplot(4,1,3); plot(scg_xyz(:,3),'b'); title('z'); box off; ylabel('Acceleration (mg)');
ax(4) = subplot(4,1,4); plot(projection,'g'); title('Mechanical Axis Projection'); box off; ylabel('Acceleration (mg)');
xlabel('Sample no.')
linkaxes(ax,'xy')
end
